simulink model "dev_switch_ekf"  (Simulink 7.0)
settings: Solver=FixedStepDiscrete  StartTime=0  StopTime=100  FixedStep=1e-3  RelTol=1e-3
undefined symbols (not defined in the file): l_fts, Q_in, R_n9, ts, zmsr
libraries: simulink x14, DLRwalkerLib x3, DLRHumanoid x2
(part 2 of 2)

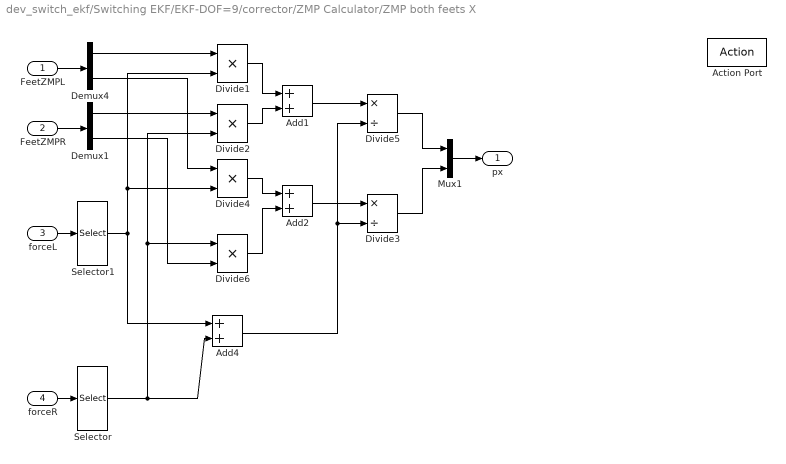
== system dev_switch_ekf/Switching EKF/EKF-DOF=9/corrector/ZMP Calculator/ZMP both feets X ==
  FeetZMPL : Inport  OutDataType=sfix(16)  OutScaling=2^0
  FeetZMPR : Inport  Port=2  OutDataType=sfix(16)  OutScaling=2^0
  forceL : Inport  Port=3  OutDataType=sfix(16)  OutScaling=2^0
  forceR : Inport  Port=4  OutDataType=sfix(16)  OutScaling=2^0
  Action Port : ActionPort  ActionType=then
  Add1 : Sum  OutDataType=sfix(16)  OutScaling=2^-10
  Add2 : Sum  OutDataType=sfix(16)  OutScaling=2^-10
  Add4 : Sum  OutDataType=sfix(16)  OutScaling=2^-10
  Demux1 : Demux  Outputs=2
  Demux4 : Demux  Outputs=2
  Divide{1..2,4,6} (4 alike) : Product  Inputs=**  OutDataType=sfix(16)  OutScaling=2^-10
  Divide3 : Product  Inputs=*/  OutDataType=sfix(16)  OutScaling=2^-10
  Divide5 : Product  Inputs=*/  OutDataType=sfix(16)  OutScaling=2^-10
  Mux1 : Mux  Inputs=2
  Selector : Selector  InputPortWidth=6  IndexOptions=Index vector (dialog)  Indices=[3]  OutputSizes=1
  Selector1 : Selector  InputPortWidth=6  IndexOptions=Index vector (dialog)  Indices=[3]  OutputSizes=1
  px : Outport  OutDataType=sfix(16)  OutScaling=2^0
  wires:
  forceR/1 -> Selector/1
  Selector/1 -> Add4/2, Divide2/2, Divide6/1
  Selector1/1 -> Add4/1, Divide1/2, Divide4/2
  forceL/1 -> Selector1/1
  Divide1/1 -> Add1/1
  Divide2/1 -> Add1/2
  Add1/1 -> Divide5/1
  Add4/1 -> Divide5/2, Divide3/2
  FeetZMPR/1 -> Demux1/1
  Demux1/1 -> Divide2/1
  FeetZMPL/1 -> Demux4/1
  Demux4/1 -> Divide1/1
  Divide4/1 -> Add2/1
  Divide6/1 -> Add2/2
  Demux4/2 -> Divide4/1
  Demux1/2 -> Divide6/2
  Add2/1 -> Divide3/1
  Mux1/1 -> px/1
  Divide5/1 -> Mux1/1
  Divide3/1 -> Mux1/2

== matlab function Switching EKF/EKF-DOF=9/predictor/Process noise ==
  data: Q_out output inherited; invT input inherited; R input inherited; Q_in input inherited
function Q_out = noise_correlation(invT,R,Q_in)
% Description : Compute the inverse of Analytical Jacobian
Z3 = zeros(3);
I3 = eye(3);
dt = 1e-3;

W = [   Z3      Z3      ;...
        Z3  -invT*dt    ;...
      -R*dt     Z3      ];
  
Q_out = W * Q_in * W';

== matlab function Switching EKF/EKF-DOF=15/predictor/Analytical Jacobian1 ==
  data: invT output inherited; o input inherited; dinvT output inherited
function [invT, dinvT] = analytical_jacobian(o)
% Description : Compute the inverse of Analytical Jacobian
o1 = o(1);
o2 = o(2);
o3 = o(3);

z = zeros(3,3);

% Rotation = Rz * Ry * Rx -----------------------------is considered
% T =
% 
% [               1,               0,        -sin(o2)]
% [               0,         cos(o1), sin(o1)*cos(o2)]
% [               0,        -sin(o1), cos(o1)*cos(o2)]

invT =[ [ 1, sin(o2)*sin(o1)/cos(o2), sin(o2)*cos(o1)/cos(o2)];...
        [ 0,                 cos(o1),                -sin(o1)];...
        [ 0,         sin(o1)/cos(o2),         cos(o1)/cos(o2)]];


dinvTdx =[[ 0,  sin(o2)*cos(o1)/cos(o2), -sin(o2)*sin(o1)/cos(o2)];...
          [ 0,                 -sin(o1),                 -cos(o1)];...
          [ 0,          cos(o1)/cos(o2),         -sin(o1)/cos(o2)]];
      
dinvTdy =[[ 0,         sin(o1)/cos(o2)^2,         cos(o1)/cos(o2)^2];...
          [ 0,                         0,                         0];...
          [ 0, sin(o1)/cos(o2)^2*sin(o2), cos(o1)/cos(o2)^2*sin(o2)]];

dinvTdz =z;

dinvT = [ dinvTdx     z        z;...
          z       dinvTdy      z;..., 
          z           z      dinvTdz ];
end

== matlab function Switching EKF/EKF-DOF=9/corrector/Eul Rotation ==
  data: g output inherited; o input inherited; dg output inherited
function [ g, dg ] = eul_rotRPY(o)
% o1 = Rotation around x 
% o2 = Rotation around y
% o3 = Rotation around z

x = o(1);
y = o(2);
z = o(3);

o1 = o(4);
o2 = o(5);
o3 = o(6);


z3 = zeros(3,3);
% This function computes the euler angles Rz*Ry*Rx
R =[
[                          cos(o3)*cos(o2), -sin(o3)*cos(o1)+cos(o3)*sin(o2)*sin(o1),  sin(o3)*sin(o1)+cos(o3)*sin(o2)*cos(o1)]
[                          sin(o3)*cos(o2),  cos(o3)*cos(o1)+sin(o3)*sin(o2)*sin(o1), -cos(o3)*sin(o1)+sin(o3)*sin(o2)*cos(o1)]
[                                 -sin(o2),                          cos(o2)*sin(o1),                          cos(o2)*cos(o1)]];

g = [ R [ x y z ]'; [ 0 0 0 1 ]];

dgdx = [ z3 [1 0 0]'; [ 0 0 0 0]];
dgdy = [ z3 [0 1 0]'; [ 0 0 0 0]];
dgdz = [ z3 [0 0 1]'; [ 0 0 0 0]];

dRdo1 = [
[                                        0,  sin(o3)*sin(o1)+cos(o3)*sin(o2)*cos(o1),  sin(o3)*cos(o1)-cos(o3)*sin(o2)*sin(o1)]
[                                        0, -cos(o3)*sin(o1)+sin(o3)*sin(o2)*cos(o1), -cos(o3)*cos(o1)-sin(o3)*sin(o2)*sin(o1)]
[                                        0,                          cos(o2)*cos(o1),                         -cos(o2)*sin(o1)]];

dgdo1 = [ dRdo1 [ 0 0 0]'; [ 0 0 0 0]]; 

dRdo2 = [
[        -cos(o3)*sin(o2), cos(o3)*cos(o2)*sin(o1), cos(o3)*cos(o2)*cos(o1)]
[        -sin(o3)*sin(o2), sin(o3)*cos(o2)*sin(o1), sin(o3)*cos(o2)*cos(o1)]
[                -cos(o2),        -sin(o2)*sin(o1),        -sin(o2)*cos(o1)]];
dgdo2 = [ dRdo2 [ 0 0 0]'; [ 0 0 0 0]]; 

dRdo3 = [
[                         -sin(o3)*cos(o2), -cos(o3)*cos(o1)-sin(o3)*sin(o2)*sin(o1),  cos(o3)*sin(o1)-sin(o3)*sin(o2)*cos(o1)]
[                          cos(o3)*cos(o2), -sin(o3)*cos(o1)+cos(o3)*sin(o2)*sin(o1),  sin(o3)*sin(o1)+cos(o3)*sin(o2)*cos(o1)]
[                                        0,                                        0,                                        0]];
dgdo3 = [ dRdo3 [ 0 0 0]'; [ 0 0 0 0]]; 

z4 = zeros(4);

dg = [ dgdx    z4    z4    z4    z4    z4;...
        z4    dgdy   z4    z4    z4    z4;...
        z4     z4   dgdz   z4    z4    z4;...
        z4     z4    z4   dgdo1  z4    z4;...
        z4     z4    z4    z4   dgdo2  z4;...
        z4     z4    z4    z4    z4   dgdo3];
% dR = [ dRdx        z        z;...
%           z       dRdy      z;... 
%           z         z      dRdz ];

== matlab function Switching EKF/EKF-DOF=15/corrector/Measurement update1 ==
  data: x_k output inherited; P output inherited; x_in input inherited; A input inherited; g_in input inherited; dg_in input inherited; kin_rf input inherited; kin_lf input inherited; cnt_msr input inherited; state input inherited; R_in input inherited; P_ input inherited; z input inherited
function [x_k,P]= fcn(x_in,A,g_in,dg_in,kin_rf, kin_lf,cnt_msr,state,R_in,P_,z)

z3 = zeros(3);

% Position of the contact points
% Contact Model:
%              b---------c
%              |      .o |          right foot
%              a---------d
%
%
%   <----      x _ _ _
%                     |            robot facing direction
%                     |
%                      y
%
%               b---------c
%               |      .o |         left foot
%               a---------d

%
% CD --> AB === Fx: 20 --> -20
% AB --> CD === Fx: -20 --> 20

contact_AB = [ 0.13 0.0475 0 1 0.13 -0.0475 0 1]';
contact_CD = [ -0.06 -0.0475 0 1 -0.06 0.0475 0 1]';

a = contact_AB(1:4);
b = contact_AB(5:8);
c = contact_CD(1:4);
d = contact_CD(5:8);
% prf = [kin_rf(1:3,4); 1];
% plf = [kin_lf(1:3,4); 1];
prfa = [kin_rf*a;1]; prfb = [kin_rf*b;1]; prfc = [kin_rf*c;1]; prfd = [kin_rf*d;1];
plfa = [kin_lf*a;1]; plfb = [kin_lf*b;1]; plfc = [kin_lf*c;1]; plfd = [kin_lf*d;1];

pra = g_in * prfa; prb = g_in * prfb; prc = g_in * prfc; prd = g_in * prfd;

pla = g_in * plfa; plb = g_in * plfb; plc = g_in * plfc; pld = g_in * plfd;

y = [pra(1:3); prb(1:3); prc(1:3); prd(1:3); pla(1:3); plb(1:3); plc(1:3); pld(1:3);];

dy = z -y;

tmp_ra = dg_in * [ prfa; prfa; prfa; prfa; prfa; prfa];
tmp_rb = dg_in * [ prfb; prfb; prfb; prfb; prfb; prfb];
tmp_rc = dg_in * [ prfc; prfc; prfc; prfc; prfc; prfc];
tmp_rd = dg_in * [ prfd; prfd; prfd; prfd; prfd; prfd];

tmp_la = dg_in * [ plfa; plfa; plfa; plfa; plfa; plfa];
tmp_lb = dg_in * [ plfb; plfb; plfb; plfb; plfb; plfb];
tmp_lc = dg_in * [ plfc; plfc; plfc; plfc; plfc; plfc];
tmp_ld = dg_in * [ plfd; plfd; plfd; plfd; plfd; plfd];

dpra = [ tmp_ra(1:3) tmp_ra(5:7) tmp_ra(9:11) tmp_ra(13:15) tmp_ra(17:19) tmp_ra(21:23) z3 z3 z3 ];
dprb = [ tmp_rb(1:3) tmp_rb(5:7) tmp_rb(9:11) tmp_rb(13:15) tmp_rb(17:19) tmp_rb(21:23) z3 z3 z3 ];
dprc = [ tmp_rc(1:3) tmp_rc(5:7) tmp_rc(9:11) tmp_rc(13:15) tmp_rc(17:19) tmp_rc(21:23) z3 z3 z3 ];
dprd = [ tmp_rd(1:3) tmp_rd(5:7) tmp_rd(9:11) tmp_rd(13:15) tmp_rd(17:19) tmp_rd(21:23) z3 z3 z3 ];
dpla = [ tmp_la(1:3) tmp_la(5:7) tmp_la(9:11) tmp_la(13:15) tmp_la(17:19) tmp_la(21:23) z3 z3 z3 ];
dplb = [ tmp_lb(1:3) tmp_lb(5:7) tmp_lb(9:11) tmp_lb(13:15) tmp_lb(17:19) tmp_lb(21:23) z3 z3 z3 ];
dplc = [ tmp_lc(1:3) tmp_lc(5:7) tmp_lc(9:11) tmp_lc(13:15) tmp_lc(17:19) tmp_lc(21:23) z3 z3 z3 ];
dpld = [ tmp_ld(1:3) tmp_ld(5:7) tmp_ld(9:11) tmp_ld(13:15) tmp_ld(17:19) tmp_ld(21:23) z3 z3 z3 ];
H = [dpra; dprb; dprc; dprd; dpla; dplb; dplc; dpld];

%%%%%%%%%%%%%%%%%%%%%%%%%%%%%%%%%%%%%%%%%MEASRUEMETN UPDATE%%%%%%%%%%%%%%%%%%%%%%%%%%%%%%%%%%%%%%%%%%%%%%%%%%%%%%%%%%%%%%%
zmp_x = cnt_msr(1); 
zmp_y = cnt_msr(2);
R = R_in;

% second foot contact pts offset
 off = 12;
K = (P_*H'/(H*P_*H'+R));
I = eye(size(P_));
P = (I-K*H)*P_*(I-K*H)' + K*R*K' ;
delx = K*dy;
if state == 2
    % Right foot support
    tmp_Hr = H(1:12,:);
    tmp_Rr = R(1:12,1:12);
    Kr = (P_*tmp_Hr'/(tmp_Hr*P_*tmp_Hr'+tmp_Rr));
    I = eye(size(P_));
    P = (I-Kr*tmp_Hr)*P_*(I-Kr*tmp_Hr)' + Kr*tmp_Rr*Kr' ;
    delx = Kr*dy(off+(1:12));
elseif state == 1
    % Left foot support
    tmp_Hl = H(off+(1:12),:);
    tmp_Rl = R(off+(1:12),off+(1:12));
    Kl = (P_*tmp_Hl'/(tmp_Hl*P_*tmp_Hl'+tmp_Rl));
    I = eye(size(P_));
    P = (I-Kl*tmp_Hl)*P_*(I-Kl*tmp_Hl)' + Kl*tmp_Rl*Kl' ;
    delx = Kl*dy(off+(1:12));
end
x_k = x_in + delx;

== matlab function Switching EKF/EKF-DOF=15/corrector/Eul Rotation ==
  data: g output inherited; o input inherited; dg output inherited
function [ g, dg ] = eul_rotRPY(o)
% o1 = Rotation around x 
% o2 = Rotation around y
% o3 = Rotation around z

x = o(1);
y = o(2);
z = o(3);

o1 = o(4);
o2 = o(5);
o3 = o(6);


z3 = zeros(3,3);
% This function computes the euler angles Rz*Ry*Rx
R =[
[                          cos(o3)*cos(o2), -sin(o3)*cos(o1)+cos(o3)*sin(o2)*sin(o1),  sin(o3)*sin(o1)+cos(o3)*sin(o2)*cos(o1)]
[                          sin(o3)*cos(o2),  cos(o3)*cos(o1)+sin(o3)*sin(o2)*sin(o1), -cos(o3)*sin(o1)+sin(o3)*sin(o2)*cos(o1)]
[                                 -sin(o2),                          cos(o2)*sin(o1),                          cos(o2)*cos(o1)]];

g = [ R [ x y z ]'; [ 0 0 0 1 ]];

dgdx = [ z3 [1 0 0]'; [ 0 0 0 0]];
dgdy = [ z3 [0 1 0]'; [ 0 0 0 0]];
dgdz = [ z3 [0 0 1]'; [ 0 0 0 0]];

dRdo1 = [
[                                        0,  sin(o3)*sin(o1)+cos(o3)*sin(o2)*cos(o1),  sin(o3)*cos(o1)-cos(o3)*sin(o2)*sin(o1)]
[                                        0, -cos(o3)*sin(o1)+sin(o3)*sin(o2)*cos(o1), -cos(o3)*cos(o1)-sin(o3)*sin(o2)*sin(o1)]
[                                        0,                          cos(o2)*cos(o1),                         -cos(o2)*sin(o1)]];

dgdo1 = [ dRdo1 [ 0 0 0]'; [ 0 0 0 0]]; 

dRdo2 = [
[        -cos(o3)*sin(o2), cos(o3)*cos(o2)*sin(o1), cos(o3)*cos(o2)*cos(o1)]
[        -sin(o3)*sin(o2), sin(o3)*cos(o2)*sin(o1), sin(o3)*cos(o2)*cos(o1)]
[                -cos(o2),        -sin(o2)*sin(o1),        -sin(o2)*cos(o1)]];
dgdo2 = [ dRdo2 [ 0 0 0]'; [ 0 0 0 0]]; 

dRdo3 = [
[                         -sin(o3)*cos(o2), -cos(o3)*cos(o1)-sin(o3)*sin(o2)*sin(o1),  cos(o3)*sin(o1)-sin(o3)*sin(o2)*cos(o1)]
[                          cos(o3)*cos(o2), -sin(o3)*cos(o1)+cos(o3)*sin(o2)*sin(o1),  sin(o3)*sin(o1)+cos(o3)*sin(o2)*cos(o1)]
[                                        0,                                        0,                                        0]];
dgdo3 = [ dRdo3 [ 0 0 0]'; [ 0 0 0 0]]; 

z4 = zeros(4);

dg = [ dgdx    z4    z4    z4    z4    z4;...
        z4    dgdy   z4    z4    z4    z4;...
        z4     z4   dgdz   z4    z4    z4;...
        z4     z4    z4   dgdo1  z4    z4;...
        z4     z4    z4    z4   dgdo2  z4;...
        z4     z4    z4    z4    z4   dgdo3];
% dR = [ dRdx        z        z;...
%           z       dRdy      z;... 
%           z         z      dRdz ];

== matlab function Switching EKF/EKF-DOF=15/predictor/Process noise ==
  data: Q_out output inherited; invT input inherited; R input inherited; Q_in input inherited
function Q_out = noise_correlation(invT,R,Q_in)
% Description : Compute the inverse of Analytical Jacobian
Z3 = zeros(3);
I3 = eye(3);
dt = 1e-3;

W = [   Z3      Z3      Z3      Z3 ;...
        Z3  -invT*dt    Z3      Z3 ;...
      -R*dt     Z3      Z3      Z3 ;...
        Z3      Z3      I3      Z3 ;...
        Z3      Z3      Z3      I3 ];

Q_out = W * Q_in * W';

== matlab function Switching EKF/EKF-DOF=15/predictor/Time Update ==
  data: A output inherited; x_k output inherited; x_in input inherited; invT input inherited; dinvT input inherited; R input inherited; dR input inherited; u_in input inherited
function [A,x_k]= fcn(x_in,invT,dinvT,R,dR,u_in)
% This block supports the Embedded MATLAB subset.
% See the help menu for details. 
dt = 1e-3;
z = zeros(3);
% x = [ pos_fb, vel_fb_s, phi, pos_rf, pos_lf ]

p = x_in(1:3);
phi = x_in(4:6);
v = x_in(7:9);
bacc = x_in(10:12);
bgyr = x_in(13:15);

% u = [ acc , ang_vel ] measured in body coordinates;
acc = u_in(1:3)-bacc;
w = u_in(4:6) - bgyr;

f = R*acc + [ 0; 0; -9.81 ] ;
p_new = p + dt*v + dt^2/2*f;
phi_new = phi + dt*invT*w;
v_new = v + dt*f;

% bias of IMU and gyro

x_k = [ p_new; phi_new;  v_new; bacc; bgyr];

% Linearization of the prediction model
%   model with 2 contact points
tmp1 = dR*[ acc; acc; acc ];
dp = [ eye(3) dt^2/2*[tmp1(1:3) tmp1(4:6) tmp1(7:9)] dt*eye(3) -dt^2/2*R z];

dv = [ z dt*[tmp1(1:3) tmp1(4:6) tmp1(7:9)] eye(3) -dt*R z];

% tmp2 = R*w;
tmp3 = dinvT*[ w ; w; w ];

dphi = [ z eye(3)+dt*[ tmp3(1:3) tmp3(4:6) tmp3(7:9) ] z z -dt*invT];
%dphi = [ z z eye(3)+dt*eye(3), z z];
A = [ dp ; dphi; dv; [zeros(6,9) eye(6)]  ];

== matlab function Switching EKF/EKF-DOF=15/predictor/Eul Rotation1 ==
  data: R output inherited; o input inherited; dR output inherited
function [ R, dR ] = eul_rotRPY(o)
% o1 = Rotation around x 
% o2 = Rotation around y
% o3 = Rotation around z 

o1 = o(1);
o2 = o(2);
o3 = o(3);


z = zeros(3,3);
% This function computes the euler angles Rz*Ry*Rx
R =[
[                          cos(o3)*cos(o2), -sin(o3)*cos(o1)+cos(o3)*sin(o2)*sin(o1),  sin(o3)*sin(o1)+cos(o3)*sin(o2)*cos(o1)]
[                          sin(o3)*cos(o2),  cos(o3)*cos(o1)+sin(o3)*sin(o2)*sin(o1), -cos(o3)*sin(o1)+sin(o3)*sin(o2)*cos(o1)]
[                                 -sin(o2),                          cos(o2)*sin(o1),                          cos(o2)*cos(o1)]];

dRdx = [
[                                        0,  sin(o3)*sin(o1)+cos(o3)*sin(o2)*cos(o1),  sin(o3)*cos(o1)-cos(o3)*sin(o2)*sin(o1)]
[                                        0, -cos(o3)*sin(o1)+sin(o3)*sin(o2)*cos(o1), -cos(o3)*cos(o1)-sin(o3)*sin(o2)*sin(o1)]
[                                        0,                          cos(o2)*cos(o1),                         -cos(o2)*sin(o1)]];

dRdy = [
[        -cos(o3)*sin(o2), cos(o3)*cos(o2)*sin(o1), cos(o3)*cos(o2)*cos(o1)]
[        -sin(o3)*sin(o2), sin(o3)*cos(o2)*sin(o1), sin(o3)*cos(o2)*cos(o1)]
[                -cos(o2),        -sin(o2)*sin(o1),        -sin(o2)*cos(o1)]];

dRdz = [
[                         -sin(o3)*cos(o2), -cos(o3)*cos(o1)-sin(o3)*sin(o2)*sin(o1),  cos(o3)*sin(o1)-sin(o3)*sin(o2)*cos(o1)]
[                          cos(o3)*cos(o2), -sin(o3)*cos(o1)+cos(o3)*sin(o2)*sin(o1),  sin(o3)*sin(o1)+cos(o3)*sin(o2)*cos(o1)]
[                                        0,                                        0,                                        0]];



% Description:
% This function computes the euler angles Rx*Ry*Rz 

% R = [
%  
% [                         cos(o2)*cos(o3),                        -cos(o2)*sin(o3),                                 sin(o2)]
% [ cos(o1)*sin(o3)+cos(o3)*sin(o1)*sin(o2), cos(o1)*cos(o3)-sin(o1)*sin(o2)*sin(o3),                        -cos(o2)*sin(o1)]
% [ sin(o1)*sin(o3)-cos(o1)*cos(o3)*sin(o2), cos(o3)*sin(o1)+cos(o1)*sin(o2)*sin(o3),                         cos(o1)*cos(o2)]];
% 
% dRdx = [
% [                                        0,                                        0,                                        0]
% [ -sin(o1)*sin(o3)+cos(o1)*cos(o3)*sin(o2), -cos(o3)*sin(o1)-cos(o1)*sin(o2)*sin(o3),                         -cos(o1)*cos(o2)]
% [  cos(o1)*sin(o3)+cos(o3)*sin(o1)*sin(o2),  cos(o1)*cos(o3)-sin(o1)*sin(o2)*sin(o3),                         -cos(o2)*sin(o1)] ];
% 
% dRdy = [ 
% [         -sin(o2)*cos(o3),          sin(o2)*sin(o3),                  cos(o2)]
% [  cos(o3)*sin(o1)*cos(o2), -sin(o1)*cos(o2)*sin(o3),          sin(o1)*sin(o2)]
% [ -cos(o1)*cos(o3)*cos(o2),  cos(o1)*cos(o2)*sin(o3),         -cos(o1)*sin(o2)]];
% 
% dRdz = [
% [                         -cos(o2)*sin(o3),                         -cos(o2)*cos(o3),                                        0]
% [  cos(o1)*cos(o3)-sin(o1)*sin(o2)*sin(o3), -cos(o1)*sin(o3)-cos(o3)*sin(o1)*sin(o2),                                        0]
% [  cos(o3)*sin(o1)+cos(o1)*sin(o2)*sin(o3), -sin(o1)*sin(o3)+cos(o1)*cos(o3)*sin(o2),                                        0]];

dR = [ dRdx        z        z;...
          z       dRdy      z;... 
          z         z      dRdz ];

== matlab function Switching EKF/EKF-DOF=15/corrector/ZMP Calculator/Embedded MATLAB Function ==
  data: enL input inherited; y output inherited; enR input inherited
function y = fcn(enL, enR)

y = 4;

if enL==1 && enR==1
    y = 3;
elseif enL==1 && enR ==0
    y = 1;
elseif enL==0 && enR ==1
    y = 2;
end

== matlab function Switching EKF/EKF-DOF=9/corrector/Measurement update1 ==
  data: x_k output inherited; P output inherited; x_in input inherited; A input inherited; g_in input inherited; dg_in input inherited; kin_rf input inherited; kin_lf input inherited; cnt_msr input inherited; state input inherited; R_in input inherited; P_ input inherited; z input inherited
function [x_k,P]= fcn(x_in,A,g_in,dg_in,kin_rf, kin_lf,cnt_msr,state,R_in,P_,z)

z3 = zeros(3);

% Position of the contact points
% Contact Model:
%              b---------c
%              |      .o |          right foot
%              a---------d
%
%
%   <----      x _ _ _
%                     |            robot facing direction
%                     |
%                      y
%
%               b---------c
%               |      .o |         left foot
%               a---------d

%
% CD --> AB === Fx: 20 --> -20
% AB --> CD === Fx: -20 --> 20

contact_AB = [ 0.13 0.0475 0 1 0.13 -0.0475 0 1]';
contact_CD = [ -0.06 -0.0475 0 1 -0.06 0.0475 0 1]';

a = contact_AB(1:4);
b = contact_AB(5:8);
c = contact_CD(1:4);
d = contact_CD(5:8);
% prf = [kin_rf(1:3,4); 1];
% plf = [kin_lf(1:3,4); 1];
prfa = [kin_rf*a;1]; prfb = [kin_rf*b;1]; prfc = [kin_rf*c;1]; prfd = [kin_rf*d;1];
plfa = [kin_lf*a;1]; plfb = [kin_lf*b;1]; plfc = [kin_lf*c;1]; plfd = [kin_lf*d;1];

pra = g_in * prfa; prb = g_in * prfb; prc = g_in * prfc; prd = g_in * prfd;

pla = g_in * plfa; plb = g_in * plfb; plc = g_in * plfc; pld = g_in * plfd;

y = [pra(1:3); prb(1:3); prc(1:3); prd(1:3); pla(1:3); plb(1:3); plc(1:3); pld(1:3);];

dy = z -y;

tmp_ra = dg_in * [ prfa; prfa; prfa; prfa; prfa; prfa];
tmp_rb = dg_in * [ prfb; prfb; prfb; prfb; prfb; prfb];
tmp_rc = dg_in * [ prfc; prfc; prfc; prfc; prfc; prfc];
tmp_rd = dg_in * [ prfd; prfd; prfd; prfd; prfd; prfd];

tmp_la = dg_in * [ plfa; plfa; plfa; plfa; plfa; plfa];
tmp_lb = dg_in * [ plfb; plfb; plfb; plfb; plfb; plfb];
tmp_lc = dg_in * [ plfc; plfc; plfc; plfc; plfc; plfc];
tmp_ld = dg_in * [ plfd; plfd; plfd; plfd; plfd; plfd];

dpra = [ tmp_ra(1:3) tmp_ra(5:7) tmp_ra(9:11) tmp_ra(13:15) tmp_ra(17:19) tmp_ra(21:23) z3];
dprb = [ tmp_rb(1:3) tmp_rb(5:7) tmp_rb(9:11) tmp_rb(13:15) tmp_rb(17:19) tmp_rb(21:23) z3];
dprc = [ tmp_rc(1:3) tmp_rc(5:7) tmp_rc(9:11) tmp_rc(13:15) tmp_rc(17:19) tmp_rc(21:23) z3];
dprd = [ tmp_rd(1:3) tmp_rd(5:7) tmp_rd(9:11) tmp_rd(13:15) tmp_rd(17:19) tmp_rd(21:23) z3];
dpla = [ tmp_la(1:3) tmp_la(5:7) tmp_la(9:11) tmp_la(13:15) tmp_la(17:19) tmp_la(21:23) z3];
dplb = [ tmp_lb(1:3) tmp_lb(5:7) tmp_lb(9:11) tmp_lb(13:15) tmp_lb(17:19) tmp_lb(21:23) z3];
dplc = [ tmp_lc(1:3) tmp_lc(5:7) tmp_lc(9:11) tmp_lc(13:15) tmp_lc(17:19) tmp_lc(21:23) z3];
dpld = [ tmp_ld(1:3) tmp_ld(5:7) tmp_ld(9:11) tmp_ld(13:15) tmp_ld(17:19) tmp_ld(21:23) z3];
H = [dpra; dprb; dprc; dprd; dpla; dplb; dplc; dpld];

%%%%%%%%%%%%%%%%%%%%%%%%%%%%%%%%%%%%%%%%%MEASRUEMETN UPDATE%%%%%%%%%%%%%%%%%%%%%%%%%%%%%%%%%%%%%%%%%%%%%%%%%%%%%%%%%%%%%%%
zmp_x = cnt_msr(1);
zmp_y = cnt_msr(2);
R = R_in;

% second foot contact pts offset
 off = 12;
% K = (P_*H'/(H*P_*H'+R));
% I = eye(size(P_));
% P = (I-K*H)*P_*(I-K*H)' + K*R*K' ;
% delx = K*dy;
if state == 3
%     % Double support or flying
    if zmp_x < -0.05 
        %rotating around back edge
        tmp_H = H([7:12 off+(7:12)],:);
        tmp_R = R([7:12 off+(7:12)],[7:12 off+(7:12)]);
        Krl = (P_*tmp_H'/(tmp_H*P_*tmp_H'+tmp_R));
        I = eye(size(P_));
        P = (I-Krl*tmp_H)*P_*(I-Krl*tmp_H)' + Krl*tmp_R*Krl' ;
        delx = Krl*dy([7:12 off+(7:12)]);

    else
        % rotating around front edge
        tmp_H = H([1:6 off+(1:6)],:);
        tmp_R = R([1:6 off+(1:6)],[1:6 off+(1:6)]);
        Krl = (P_*tmp_H'/(tmp_H*P_*tmp_H'+tmp_R));
        I = eye(size(P_));
        P = (I-Krl*tmp_H)*P_*(I-Krl*tmp_H)' + Krl*tmp_R*Krl' ;
        delx = Krl*dy([1:6 off+(1:6)]);
    end

elseif state == 2
    % Support Right foot
    if zmp_y < -0.0375
        % Tilting around outer edge
        tmp_Hr = H(4:9,:);
        tmp_Rr = R(4:9,4:9);
        Kr = (P_*tmp_Hr'/(tmp_Hr*P_*tmp_Hr'+tmp_Rr));
        I = eye(size(P_));
        P = (I-Kr*tmp_Hr)*P_*(I-Kr*tmp_Hr)' + Kr*tmp_Rr*Kr' ;
        delx = Kr*dy(4:9);
    else
        %Tilting around inner edge
        tmp_Hr = H([1:3 10:12],:);
        tmp_Rr = R([1:3 10:12],[1:3 10:12]);
        Kr = (P_*tmp_Hr'/(tmp_Hr*P_*tmp_Hr'+tmp_Rr));
        I = eye(size(P_));
        P = (I-Kr*tmp_Hr)*P_*(I-Kr*tmp_Hr)' + Kr*tmp_Rr*Kr' ;
        delx = Kr*dy([1:3 10:12]);
    end
    
else
    % Support Left foot
    if zmp_y < -0.0375
        % Tilting around inner edge
        tmp_Hl = H(off+(4:9),:);
        tmp_Rl = R(off+(4:9),off+(4:9));
        Kl = (P_*tmp_Hl'/(tmp_Hl*P_*tmp_Hl'+tmp_Rl));
        I = eye(size(P_));
        P = (I-Kl*tmp_Hl)*P_*(I-Kl*tmp_Hl)' + Kl*tmp_Rl*Kl' ;
        delx = Kl*dy(off+(4:9));
    else
        %Tilting around outer edge
        tmp_Hl = H([ off+(1:3) off+(10:12)],:);
        tmp_Rl = R([off+(1:3) off+(10:12)],[off+(1:3) off+(10:12)]);
        Kl = (P_*tmp_Hl'/(tmp_Hl*P_*tmp_Hl'+tmp_Rl));
        I = eye(size(P_));
        P = (I-Kl*tmp_Hl)*P_*(I-Kl*tmp_Hl)' + Kl*tmp_Rl*Kl' ;
        delx = Kl*dy([off+(1:3) off+(10:12)]);
    end
end
x_k = x_in + delx;

== matlab function Switching EKF/EKF-DOF=9/corrector/ZMP Calculator/Embedded MATLAB Function ==
  data: enL input inherited; y output inherited; enR input inherited
function y = fcn(enL, enR)

y = 4;

if enL==1 && enR==1
    y = 3;
elseif enL==1 && enR ==0
    y = 1;
elseif enL==0 && enR ==1
    y = 2;
end

== matlab function Switching EKF/Subsystem/ZMP Calculator/Embedded MATLAB Function ==
  data: enL input inherited; y output inherited; enR input inherited
function y = fcn(enL, enR)

y = 4;

if enL==1 && enR==1
    y = 3;
elseif enL==1 && enR ==0
    y = 1;
elseif enL==0 && enR ==1
    y = 2;
end

== matlab function Switching EKF/EKF-DOF=9/predictor/Analytical Jacobian1 ==
  data: invT output inherited; o input inherited; dinvT output inherited
function [invT, dinvT] = analytical_jacobian(o)
% Description : Compute the inverse of Analytical Jacobian
o1 = o(1);
o2 = o(2);
o3 = o(3);

z = zeros(3,3);

% Rotation = Rz * Ry * Rx -----------------------------is considered
% T =
% 
% [               1,               0,        -sin(o2)]
% [               0,         cos(o1), sin(o1)*cos(o2)]
% [               0,        -sin(o1), cos(o1)*cos(o2)]

invT =[ [ 1, sin(o2)*sin(o1)/cos(o2), sin(o2)*cos(o1)/cos(o2)];...
        [ 0,                 cos(o1),                -sin(o1)];...
        [ 0,         sin(o1)/cos(o2),         cos(o1)/cos(o2)]];


dinvTdx =[[ 0,  sin(o2)*cos(o1)/cos(o2), -sin(o2)*sin(o1)/cos(o2)];...
          [ 0,                 -sin(o1),                 -cos(o1)];...
          [ 0,          cos(o1)/cos(o2),         -sin(o1)/cos(o2)]];
      
dinvTdy =[[ 0,         sin(o1)/cos(o2)^2,         cos(o1)/cos(o2)^2];...
          [ 0,                         0,                         0];...
          [ 0, sin(o1)/cos(o2)^2*sin(o2), cos(o1)/cos(o2)^2*sin(o2)]];

dinvTdz =z;

dinvT = [ dinvTdx     z        z;...
          z       dinvTdy      z;..., 
          z           z      dinvTdz ];
end

== matlab function Switching EKF/EKF-DOF=9/predictor/Eul Rotation1 ==
  data: R output inherited; o input inherited; dR output inherited
function [ R, dR ] = eul_rotRPY(o)
% o1 = Rotation around x 
% o2 = Rotation around y
% o3 = Rotation around z

o1 = o(1);
o2 = o(2);
o3 = o(3);


z = zeros(3,3);
% This function computes the euler angles Rz*Ry*Rx
R =[
[                          cos(o3)*cos(o2), -sin(o3)*cos(o1)+cos(o3)*sin(o2)*sin(o1),  sin(o3)*sin(o1)+cos(o3)*sin(o2)*cos(o1)]
[                          sin(o3)*cos(o2),  cos(o3)*cos(o1)+sin(o3)*sin(o2)*sin(o1), -cos(o3)*sin(o1)+sin(o3)*sin(o2)*cos(o1)]
[                                 -sin(o2),                          cos(o2)*sin(o1),                          cos(o2)*cos(o1)]];

dRdx = [
[                                        0,  sin(o3)*sin(o1)+cos(o3)*sin(o2)*cos(o1),  sin(o3)*cos(o1)-cos(o3)*sin(o2)*sin(o1)]
[                                        0, -cos(o3)*sin(o1)+sin(o3)*sin(o2)*cos(o1), -cos(o3)*cos(o1)-sin(o3)*sin(o2)*sin(o1)]
[                                        0,                          cos(o2)*cos(o1),                         -cos(o2)*sin(o1)]];

dRdy = [
[        -cos(o3)*sin(o2), cos(o3)*cos(o2)*sin(o1), cos(o3)*cos(o2)*cos(o1)]
[        -sin(o3)*sin(o2), sin(o3)*cos(o2)*sin(o1), sin(o3)*cos(o2)*cos(o1)]
[                -cos(o2),        -sin(o2)*sin(o1),        -sin(o2)*cos(o1)]];

dRdz = [
[                         -sin(o3)*cos(o2), -cos(o3)*cos(o1)-sin(o3)*sin(o2)*sin(o1),  cos(o3)*sin(o1)-sin(o3)*sin(o2)*cos(o1)]
[                          cos(o3)*cos(o2), -sin(o3)*cos(o1)+cos(o3)*sin(o2)*sin(o1),  sin(o3)*sin(o1)+cos(o3)*sin(o2)*cos(o1)]
[                                        0,                                        0,                                        0]];



% Description:
% This function computes the euler angles Rx*Ry*Rz 

% R = [
%  
% [                         cos(o2)*cos(o3),                        -cos(o2)*sin(o3),                                 sin(o2)]
% [ cos(o1)*sin(o3)+cos(o3)*sin(o1)*sin(o2), cos(o1)*cos(o3)-sin(o1)*sin(o2)*sin(o3),                        -cos(o2)*sin(o1)]
% [ sin(o1)*sin(o3)-cos(o1)*cos(o3)*sin(o2), cos(o3)*sin(o1)+cos(o1)*sin(o2)*sin(o3),                         cos(o1)*cos(o2)]];
% 
% dRdx = [
% [                                        0,                                        0,                                        0]
% [ -sin(o1)*sin(o3)+cos(o1)*cos(o3)*sin(o2), -cos(o3)*sin(o1)-cos(o1)*sin(o2)*sin(o3),                         -cos(o1)*cos(o2)]
% [  cos(o1)*sin(o3)+cos(o3)*sin(o1)*sin(o2),  cos(o1)*cos(o3)-sin(o1)*sin(o2)*sin(o3),                         -cos(o2)*sin(o1)] ];
% 
% dRdy = [ 
% [         -sin(o2)*cos(o3),          sin(o2)*sin(o3),                  cos(o2)]
% [  cos(o3)*sin(o1)*cos(o2), -sin(o1)*cos(o2)*sin(o3),          sin(o1)*sin(o2)]
% [ -cos(o1)*cos(o3)*cos(o2),  cos(o1)*cos(o2)*sin(o3),         -cos(o1)*sin(o2)]];
% 
% dRdz = [
% [                         -cos(o2)*sin(o3),                         -cos(o2)*cos(o3),                                        0]
% [  cos(o1)*cos(o3)-sin(o1)*sin(o2)*sin(o3), -cos(o1)*sin(o3)-cos(o3)*sin(o1)*sin(o2),                                        0]
% [  cos(o3)*sin(o1)+cos(o1)*sin(o2)*sin(o3), -sin(o1)*sin(o3)+cos(o1)*cos(o3)*sin(o2),                                        0]];

dR = [ dRdx        z        z;...
          z       dRdy      z;... 
          z         z      dRdz ];

== matlab function Switching EKF/EKF-DOF=9/predictor/Time Update ==
  data: A output inherited; x_k output inherited; x_in input inherited; b_in input inherited; invT input inherited; dinvT input inherited; R input inherited; dR input inherited; u_in input inherited
function [A,x_k]= fcn(x_in,b_in,invT,dinvT,R,dR,u_in)
% This block supports the Embedded MATLAB subset.
% See the help menu for details. 
dt = 1e-3;
z = zeros(3);
% x = [ pos_fb, vel_fb_s, phi, pos_rf, pos_lf ]

p = x_in(1:3);
phi = x_in(4:6);
v = x_in(7:9);
bacc = b_in(1:3);
bgyr = b_in(4:6);

% u = [ acc , ang_vel ] measured in body coordinates;
acc = u_in(1:3)-bacc;
w = u_in(4:6) - bgyr;

f = R*acc + [ 0; 0; -9.81 ] ;
p_new = p + dt*v + dt^2/2*f;
phi_new = phi + dt*invT*w;
v_new = v + dt*f;

% bias of IMU and gyro

x_k = [ p_new; phi_new;  v_new];

% Linearization of the prediction model
%   model with 2 contact points
tmp1 = dR*[ acc; acc; acc ];
dp = [ eye(3) dt^2/2*[tmp1(1:3) tmp1(4:6) tmp1(7:9)] dt*eye(3)];

dv = [ z dt*[tmp1(1:3) tmp1(4:6) tmp1(7:9)] eye(3)];
tmp3 = dinvT*[ w ; w; w ];
dphi = [ z eye(3)+dt*[ tmp3(1:3) tmp3(4:6) tmp3(7:9) ] z];
%dphi = [ z z eye(3)+dt*eye(3), z z];
A = [ dp ; dphi; dv ];

== matlab function Switching EKF/Subsystem/conact ==
  data: y output inherited; zmp input inherited; state input inherited
function y  = contact_switch(zmp,state)
zmp_x = zmp(1);
zmp_y = zmp(2);

if state == 3
    % Double support
    if zmp_x < -0.05 || zmp_x > 0.12
        % Rotating around y axis
        y = 1;
    else
        y = 2;
    end
elseif state == 2 || state == 1
    % Single Support
    if zmp_y < -0.04 || zmp_y > 0.04 || zmp_x < -0.05 || zmp_x > 0.12
        % Tilting around one axis
        y = 1;
    else
        y = 2;
    end
else    
        y = 2;
end

== matlab function Switching EKF/EKF-DOF=9/conact ==
  data: P_k output inherited; P_in input inherited; P_out input inherited
function P_k  = contact_switch(P_in,P_out)
tmp_Pin = P_in;
tmp_Pin(1:9,1:9) = zeros(9);

tmp_Pout = zeros(size(P_in));
tmp_Pout(1:9,1:9) = P_out;

P_k = tmp_Pin + tmp_Pout ;
